simulink model "estModel"  (R2017a)
settings: Solver=FixedStepAuto  StartTime=0.0  StopTime=simTime  FixedStep=0.1  RelTol=1e-3
values from neighbouring files (symbols this model uses):
  dt = 0.1    [exmM_IM.m]
undefined symbols (not defined in the file or in its folder): idss
libraries: slident x1
settings Model: Creator=lzr96  LastModifiedBy=lzr96

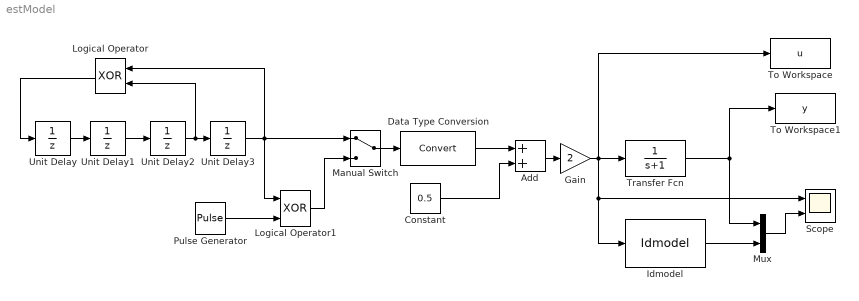
== system estModel ==
  Add : Sum
  Constant : Constant  Value=0.5
  Data Type Conversion : DataTypeConversion
  Gain : Gain  Gain=2
  Idmodel : slident/Models/Idmodel  sys=idss(-1,1,1,0,'Ts',1)  IC=0  noi=on  seed=[]
      settings: SourceProductName=System Identification Toolbox  SourceProductBaseCode=ID
  Logical Operator : Logic  Operator=XOR  AllPortsSameDT=off  OutDataTypeStr=boolean
  Logical Operator1 : Logic  Operator=XOR  AllPortsSameDT=off  OutDataTypeStr=boolean
  Manual Switch : ManualSwitch
  Mux : Mux  Inputs=2
  Pulse Generator : DiscretePulseGenerator  PulseType=Time based  Period=dt*2  PulseWidth=50
  Scope : Scope  NumInputPorts=2
  To Workspace : ToWorkspace  VariableName=u  SampleTime=-1
  To Workspace1 : ToWorkspace  VariableName=y  SampleTime=-1
  Transfer Fcn : TransferFcn  Denominator=[1 1]
  Unit Delay : UnitDelay  InitialCondition=1  SampleTime=-1
  Unit Delay1 : UnitDelay  SampleTime=-1
  Unit Delay2 : UnitDelay  SampleTime=-1
  Unit Delay3 : UnitDelay  SampleTime=-1
  wires:
  Unit Delay3/1 -> Logical Operator/1, Manual Switch/1, Logical Operator1/1
  Unit Delay/1 -> Unit Delay1/1
  Constant/1 -> Add/2
  Add/1 -> Gain/1
  Unit Delay1/1 -> Unit Delay2/1
  Unit Delay2/1 -> Logical Operator/2, Unit Delay3/1
  Logical Operator/1 -> Unit Delay/1
  Data Type Conversion/1 -> Add/1
  Gain/1 -> To Workspace/1, Scope/1, Idmodel/1, Transfer Fcn/1
  Manual Switch/1 -> Data Type Conversion/1
  Pulse Generator/1 -> Logical Operator1/2
  Logical Operator1/1 -> Manual Switch/2
  Transfer Fcn/1 -> Mux/1, To Workspace1/1
  Idmodel/1 -> Mux/2
  Mux/1 -> Scope/2
